simulink model "model_with_function_block"  (R2024b)
settings: Solver=ode45  StartTime=0.0  StopTime=100  MaxStep=0.01  RelTol=1e-3  AbsTol=1e-3  EnableMultiTasking=on
values from neighbouring files (symbols this model uses):
  a = 0.2359    [parameters.m]
  B = 14.17    [parameters.m]
  c = 0.95e3    (= 950)    [parameters.m]
  C = 1.85    [parameters.m]
  D = 1    [parameters.m]
  E = 0.97    [parameters.m]
  g = 9.81    [parameters.m]
  h = 0.2057    [parameters.m]
  h0 = 0.35    [parameters.m]
  J_Cx = m*(4*w^2+4*h^2)/6    (= 553.66011914)    [parameters.m]
  J_Cy = m*(l^2+4*h^2)/6    (= 2106.98496914)    [parameters.m]
  J_Cz = m*(l^2+4*w^2)/6    (= 2611.05485)    [parameters.m]
  k = 30e3    (= 30000)    [parameters.m]
  l = 3.77    [parameters.m]
  m = 879    [parameters.m]
  m_small = 1e-3    (= 0.001)    [parameters.m]
  v = 20    [parameters.m]
  w = 0.95    [parameters.m]
undefined symbols (not defined in the file or in its folder): X, Y, Z
libraries: sm_lib x37, nesl_utility x12
(part 2 of 2)

== matlab function model_with_function_block/MATLAB Function1 ==
  data: z input; FtireR output; FtireL output; param input
function [FtireR, FtireL] = trailer_tireforces(z,param)

	% state variables
	psi = z(1,1);
	theta = z(2,1);
	fi = z(3,1);
	u = z(4,1);
	psid = z(5,1);
	thetad = z(6,1);
	fid = z(7,1);
	ud = z(8,1);
    
	
	% parameters  
	eps = 1e-3;

	g = param(1); 
    l = param(2);
    w = param(3);
    h0 = param(4);
    a = param(5);
    m = param(6);
    k = param(7);
    c = param(8);
    B = param(9);
    C = param(10);
    D = param(11);
    E = param(12);
    v = param(13);
	

    

	LB0 = h0+m*g*(l-a)/(2*k*l);
	%LB0 = 0.0474; % experimental rig
    
	LJ0 = LB0;
	lambdaTB = 1/cos(fi)*(h0/cos(theta)+w*sin(fi)+l*tan(theta));
	lambdaTJ = 1/cos(fi)*(h0/cos(theta)-w*sin(fi)+l*tan(theta));
	
	j3R0XY = [-(cos(fi)*sin(psi))+cos(psi)*sin(fi)*sin(theta);cos(fi)*cos(psi)+sin(fi)*sin(psi)*sin(theta);0];
	ylat = j3R0XY/norm(j3R0XY);
	% xh = [-ylat(2); ylat(1); ylat(3)];
	
	vTBR0 = [v-w*psid*cos(fi)*cos(psi)+l*psid*cos(theta)*sin(psi)-h0*psid*cos(psi)*1/cos(theta)*tan(fi)-w*psid*cos(psi)*sin(fi)*tan(fi)-thetad*1/cos(theta)^2*(cos(psi)*(h0+l*sin(theta))+sin(psi)*(l+h0*sin(theta))*tan(fi))+h0*psid*sin(psi)*tan(theta)+l*psid*sin(psi)*sin(theta)*tan(theta)-l*psid*cos(psi)*tan(fi)*tan(theta)-fid*1/cos(fi)^2*sin(psi)*(h0*1/cos(theta)+w*sin(fi)+l*tan(theta));
    	ud-l*psid*cos(psi)*cos(theta)+fid*h0*cos(psi)*1/cos(theta)+w*fid*cos(psi)*sin(fi)-w*psid*cos(fi)*sin(psi)-h0*psid*1/cos(theta)*sin(psi)*tan(fi)-w*psid*sin(fi)*sin(psi)*tan(fi)+fid*h0*cos(psi)*1/cos(theta)*tan(fi)^2+w*fid*cos(psi)*sin(fi)*tan(fi)^2-thetad*1/cos(theta)^2*(sin(psi)*(h0+l*sin(theta))-cos(psi)*(l+h0*sin(theta))*tan(fi))+fid*l*cos(psi)*tan(theta)-h0*psid*cos(psi)*tan(theta)-l*psid*cos(psi)*sin(theta)*tan(theta)-l*psid*sin(psi)*tan(fi)*tan(theta)+fid*l*cos(psi)*tan(fi)^2*tan(theta);
    	0];
	vTJR0 = [v+w*psid*cos(fi)*cos(psi)+l*psid*cos(theta)*sin(psi)-h0*psid*cos(psi)*1/cos(theta)*tan(fi)+w*psid*cos(psi)*sin(fi)*tan(fi)-thetad*1/cos(theta)^2*(cos(psi)*(h0+l*sin(theta))+sin(psi)*(l+h0*sin(theta))*tan(fi))+h0*psid*sin(psi)*tan(theta)+l*psid*sin(psi)*sin(theta)*tan(theta)-l*psid*cos(psi)*tan(fi)*tan(theta)-fid*1/cos(fi)^2*sin(psi)*(h0*1/cos(theta)-w*sin(fi)+l*tan(theta));
    	ud-l*psid*cos(psi)*cos(theta)+fid*h0*cos(psi)*1/cos(theta)-w*fid*cos(psi)*sin(fi)+w*psid*cos(fi)*sin(psi)-h0*psid*1/cos(theta)*sin(psi)*tan(fi)+w*psid*sin(fi)*sin(psi)*tan(fi)+fid*h0*cos(psi)*1/cos(theta)*tan(fi)^2-w*fid*cos(psi)*sin(fi)*tan(fi)^2-thetad*1/cos(theta)^2*(sin(psi)*(h0+l*sin(theta))-cos(psi)*(l+h0*sin(theta))*tan(fi))+fid*l*cos(psi)*tan(theta)-h0*psid*cos(psi)*tan(theta)-l*psid*cos(psi)*sin(theta)*tan(theta)-l*psid*sin(psi)*tan(fi)*tan(theta)+fid*l*cos(psi)*tan(fi)^2*tan(theta);
    	0];

	vTBR3 = [(v*cos(psi)*cos(theta)-w*psid*cos(theta)*1/cos(fi)+v*cos(psi)*1/cos(theta)-w*psid*1/cos(fi)*1/cos(theta)+2*ud*cos(theta)*sin(psi)-2*thetad*1/cos(theta)*(h0+l*sin(theta))-2*h0*psid*tan(fi)-2*l*psid*sin(theta)*tan(fi)-v*cos(psi)*sin(theta)*tan(theta)+w*psid*1/cos(fi)*sin(theta)*tan(theta))/2;
    ud*(cos(fi)*cos(psi)+sin(fi)*sin(psi)*sin(theta))+(-(l*psid*cos(fi)*cos(theta))+l*psid*cos(theta)*1/cos(fi)-l*psid*cos(fi)*1/cos(theta)-3*l*psid*1/cos(fi)*1/cos(theta)+4*l*thetad*sin(fi)-2*v*cos(fi)*sin(psi)-2*v*1/cos(fi)*sin(psi)+4*v*cos(psi)*sin(fi)*sin(theta)+l*psid*cos(theta)*sin(fi)*tan(fi)+l*psid*1/cos(theta)*sin(fi)*tan(fi)+2*v*sin(fi)*sin(psi)*tan(fi)-4*w*psid*sin(theta)*tan(fi)-4*h0*psid*1/cos(fi)*tan(theta)+l*psid*cos(fi)*sin(theta)*tan(theta)-l*psid*1/cos(fi)*sin(theta)*tan(theta)-l*psid*sin(fi)*sin(theta)*tan(fi)*tan(theta)+4*fid*(h0*1/cos(fi)*1/cos(theta)+w*tan(fi)+l*1/cos(fi)*tan(theta)))/4;
    ud*(-(cos(psi)*sin(fi))+cos(fi)*sin(psi)*sin(theta))+(thetad*1/cos(fi)*1/cos(theta)^2*(-6*l+2*l*cos(2*fi)+2*l*cos(2*theta)+l*cos(2*(-fi+theta))+l*cos(2*(fi+theta))-8*h0*sin(theta))+8*(l*psid*cos(theta)*sin(fi)+v*sin(fi)*sin(psi)-w*psid*sin(theta)+v*cos(fi)*cos(psi)*sin(theta)-fid*1/cos(fi)*tan(fi)*(h0*1/cos(theta)+w*sin(fi)+l*tan(theta))))/8];
	vTJR3 = [(v*cos(psi)*cos(theta)+w*psid*cos(theta)*1/cos(fi)+v*cos(psi)*1/cos(theta)+w*psid*1/cos(fi)*1/cos(theta)+2*ud*cos(theta)*sin(psi)-2*thetad*1/cos(theta)*(h0+l*sin(theta))-2*h0*psid*tan(fi)-2*l*psid*sin(theta)*tan(fi)-v*cos(psi)*sin(theta)*tan(theta)-w*psid*1/cos(fi)*sin(theta)*tan(theta))/2;
    ud*(cos(fi)*cos(psi)+sin(fi)*sin(psi)*sin(theta))+(-(l*psid*cos(fi)*cos(theta))+l*psid*cos(theta)*1/cos(fi)-l*psid*cos(fi)*1/cos(theta)-3*l*psid*1/cos(fi)*1/cos(theta)+4*l*thetad*sin(fi)-2*v*cos(fi)*sin(psi)-2*v*1/cos(fi)*sin(psi)+4*v*cos(psi)*sin(fi)*sin(theta)+l*psid*cos(theta)*sin(fi)*tan(fi)+l*psid*1/cos(theta)*sin(fi)*tan(fi)+2*v*sin(fi)*sin(psi)*tan(fi)+4*w*psid*sin(theta)*tan(fi)-4*h0*psid*1/cos(fi)*tan(theta)+l*psid*cos(fi)*sin(theta)*tan(theta)-l*psid*1/cos(fi)*sin(theta)*tan(theta)-l*psid*sin(fi)*sin(theta)*tan(fi)*tan(theta)+4*fid*(h0*1/cos(fi)*1/cos(theta)-w*tan(fi)+l*1/cos(fi)*tan(theta)))/4;
    ud*(-(cos(psi)*sin(fi))+cos(fi)*sin(psi)*sin(theta))+(thetad*1/cos(fi)*1/cos(theta)^2*(-6*l+2*l*cos(2*fi)+2*l*cos(2*theta)+l*cos(2*(-fi+theta))+l*cos(2*(fi+theta))-8*h0*sin(theta))+8*(l*psid*cos(theta)*sin(fi)+v*sin(fi)*sin(psi)+w*psid*sin(theta)+v*cos(fi)*cos(psi)*sin(theta)-fid*1/cos(fi)*tan(fi)*(h0*1/cos(theta)-w*sin(fi)+l*tan(theta))))/8];

	vBR3 = [(-(w*psid*cos(fi))+v*cos(psi))*cos(theta)+w*thetad*sin(fi)+ud*cos(theta)*sin(psi);
    -(l*psid*cos(fi)*cos(theta))+l*thetad*sin(fi)-v*cos(fi)*sin(psi)+v*cos(psi)*sin(fi)*sin(theta)+ud*(cos(fi)*cos(psi)+sin(fi)*sin(psi)*sin(theta));
    w*fid+l*thetad*cos(fi)+l*psid*cos(theta)*sin(fi)+v*sin(fi)*sin(psi)-w*psid*sin(theta)+v*cos(fi)*cos(psi)*sin(theta)+ud*(-(cos(psi)*sin(fi))+cos(fi)*sin(psi)*sin(theta))];
	vJR3 = [(w*psid*cos(fi)+v*cos(psi))*cos(theta)-w*thetad*sin(fi)+ud*cos(theta)*sin(psi);
    -(l*psid*cos(fi)*cos(theta))+l*thetad*sin(fi)-v*cos(fi)*sin(psi)+v*cos(psi)*sin(fi)*sin(theta)+ud*(cos(fi)*cos(psi)+sin(fi)*sin(psi)*sin(theta));
    -(w*fid)+l*thetad*cos(fi)+l*psid*cos(theta)*sin(fi)+v*sin(fi)*sin(psi)+w*psid*sin(theta)+v*cos(fi)*cos(psi)*sin(theta)+ud*(-(cos(psi)*sin(fi))+cos(fi)*sin(psi)*sin(theta))];

	
	alfaB = -atan(vTBR0'*ylat/sqrt((vTBR0-(vTBR0'*ylat)*ylat)'*(vTBR0-(vTBR0'*ylat)*ylat)));
	alfaJ = -atan(vTJR0'*ylat/sqrt((vTJR0-(vTJR0'*ylat)*ylat)'*(vTJR0-(vTJR0'*ylat)*ylat)));
	
	srugoInf = 2*k;
	kcsillInf= 2*c;
	
	% forces in the suspension system, bh=lh (corrected)
	FBrugo10 = (LB0-lambdaTB)*k+(vTBR3(3)-vBR3(3))*c;
	FBrugo20 = (-lambdaTB)*srugoInf+(vTBR3(3)-vBR3(3))*kcsillInf;
	% FBrugo = (FBrugo10*(1+tanh((LB0-p-lambdaTB)/eps))/2+FBrugo20*(1+tanh((lh-lambdaTB)/eps))/2)*(1+tanh(FBrugo10/eps))/2;
	% with the correct ReLU function:
   
	FBrugo = (FBrugo10*(1+tanh((LB0-lambdaTB)/eps))/2+FBrugo20*(1+tanh((-lambdaTB)/eps))/2)*(1+tanh((FBrugo10*(1+tanh((LB0-lambdaTB)/eps))/2+FBrugo20*(1+tanh((-lambdaTB)/eps))/2)/eps))/2;
	
	FJrugo10 = (LJ0-lambdaTJ)*k+(vTJR3(3)-vJR3(3))*c;
	FJrugo20 = (-lambdaTJ)*srugoInf+(vTJR3(3)-vJR3(3))*kcsillInf;
	% FJrugo = (FJrugo10*(1+tanh((LJ0-p-lambdaTJ)/eps))/2+FJrugo20*(1+tanh((lh-lambdaTJ)/eps))/2)*(1+tanh(FJrugo10/eps))/2;
	% with the correct ReLU function:
	FJrugo = (FJrugo10*(1+tanh((LJ0-lambdaTJ)/eps))/2+FJrugo20*(1+tanh((-lambdaTJ)/eps))/2)*(1+tanh((FJrugo10*(1+tanh((LJ0-lambdaTJ)/eps))/2+FJrugo20*(1+tanh((-lambdaTJ)/eps))/2)/eps))/2;
        	
	FTBZ0 = FBrugo*cos(fi)*cos(theta);
	FTJZ0 = FJrugo*cos(fi)*cos(theta);
	
	% Magic Formula
	% B = 14.1737; C = 1.84633; D = 1; E = 0.97; % Darling 
    muB=D*sin(C*atan(B*alfaB-E*(B*alfaB-atan(B*alfaB))));
	FBtyre = FTBZ0*muB;
    muJ=D*sin(C*atan(B*alfaJ-E*(B*alfaJ-atan(B*alfaJ))));
	FJtyre = FTJZ0*muJ;
    FtireL = FBtyre*ylat;
    FtireR = FJtyre*ylat;


end
